simulink model "NEDC_Profiles"  (R2021b)
settings: Solver=VariableStepAuto  StartTime=0.0  StopTime=1190  RelTol=1e-3
undefined symbols (not defined in the file or in its folder): S_CYCLE, T_CYCLE, T_MAX
libraries: simulink x1
settings Model: Creator=Alireza  LastModifiedBy=Alireza

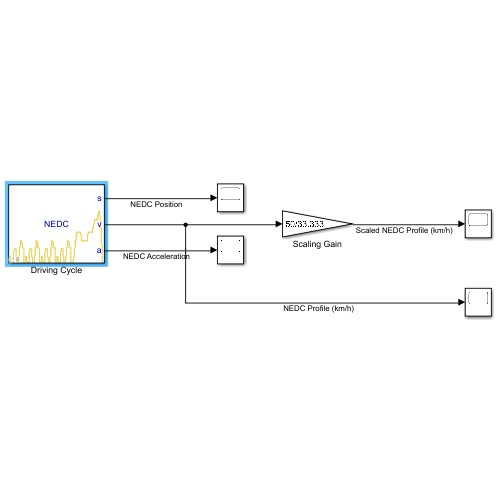
[thumbnail: Simulink's stored preview of the top-level diagram]
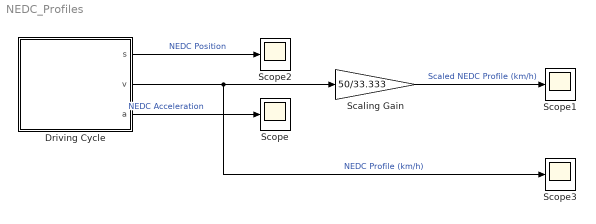
== system NEDC_Profiles ==
  Driving Cycle : Subsystem  AncestorBlock=drivingcycle_lib/Driving Cycle  mask(Driving Cycle){CycleName=NEDC, CycleRepeatsForever=off}
      mask prompts: CycleName "Cycle name:"; CycleRepeatsForever "Repeat cycle forever"
      mask help: This block produces driving cycle data, as used in many automotive applications. It outputs displacement, velocity and acceleration, all in SI units. The user can choose from a list of popular cycles.
      mask init:
      | [S_CYCLE, T_CYCLE, T_MAX, W_SCALE, Disp, Vel, Acc, t, v] = ...
      |     drivingcycleutils.maskInitFcn(CycleName, CycleRepeatsForever);
      mask Help: web(drivingcycleutils.docPath(gcb()), '-helpbrowser');
      mask TypeOptions CycleName: NEDC | ECE R15 | EUDC | ArtUrban | ArtRoad | ArtMw130 | ArtMw150 | WLTP class 3 | UDDS | FTP | HWFET
      mask Display:
      | color('yellow');
      | plot(t/max(t),3.6*v/180);
      | color('blue')
      | fprintf(CycleName);
      | port_label('output', 1, 's');
      | port_label('output', 2, 'v');
      | port_label('output', 3, 'a');
  Scaling Gain : Gain  Gain=50/33.333
  Scope{,1..3} (4 alike) : Scope
  wires:
  Driving Cycle/2(v) -> Scope3/1, Scaling Gain/1  "NEDC Profile (km/h)"
  Driving Cycle/3(a) -> Scope/1  "NEDC Acceleration"
  Scaling Gain/1 -> Scope1/1  "Scaled NEDC Profile (km/h)"
  Driving Cycle/1(s) -> Scope2/1  "NEDC Position"

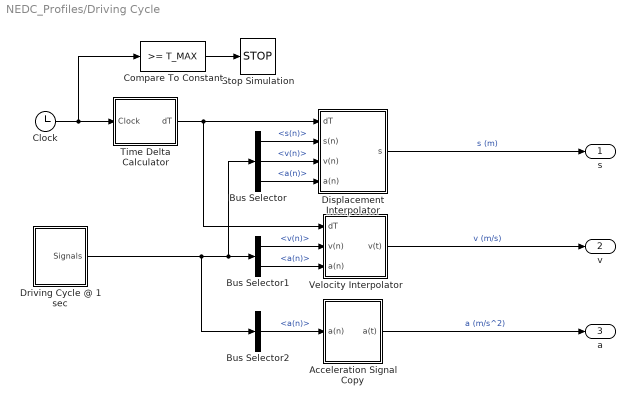
== system NEDC_Profiles/Driving Cycle ==
  Acceleration Signal Copy : Subsystem
  Bus Selector : BusSelector  OutputSignals=s(n),v(n),a(n)
  Bus Selector1 : BusSelector  OutputSignals=v(n),a(n)
  Bus Selector2 : BusSelector  OutputSignals=a(n)
  Clock : Clock
  Compare To Constant : simulink/Logic and Bit Operations/Compare To Constant  relop=>=  const=T_MAX  OutDataTypeStr=boolean
  Displacement Interpolator : Subsystem
  Driving Cycle @ 1 sec : Subsystem
  Stop Simulation : Stop
  Time Delta Calculator : Subsystem
  Velocity Interpolator : Subsystem
  s : Outport
  v : Outport  Port=2
  a : Outport  Port=3
  wires:
  Compare To Constant/1 -> Stop Simulation/1
  Time Delta Calculator/1(dT) -> Displacement Interpolator/1(dT), Velocity Interpolator/1(dT)
  Displacement Interpolator/1(s) -> s/1  "s (m)"
  Velocity Interpolator/1(v(t)) -> v/1  "v (m/s)"
  Driving Cycle @ 1 sec/1(Signals) -> Bus Selector/1, Bus Selector1/1, Bus Selector2/1
  Bus Selector/1 -> Displacement Interpolator/2(s(n))  "<s(n)>"
  Bus Selector/2 -> Displacement Interpolator/3(v(n))  "<v(n)>"
  Bus Selector/3 -> Displacement Interpolator/4(a(n))  "<a(n)>"
  Bus Selector1/1 -> Velocity Interpolator/2(v(n))  "<v(n)>"
  Bus Selector1/2 -> Velocity Interpolator/3(a(n))  "<a(n)>"
  Bus Selector2/1 -> Acceleration Signal Copy/1(a(n))  "<a(n)>"
  Acceleration Signal Copy/1(a(t)) -> a/1  "a (m/s^2)"
  Clock/1 -> Compare To Constant/1, Time Delta Calculator/1(Clock)

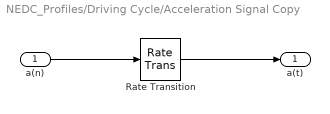
== system NEDC_Profiles/Driving Cycle/Acceleration Signal Copy ==
  a(n) : Inport
  Rate Transition : RateTransition  Integrity=off
  a(t) : Outport
  wires:
  a(n)/1 -> Rate Transition/1
  Rate Transition/1 -> a(t)/1

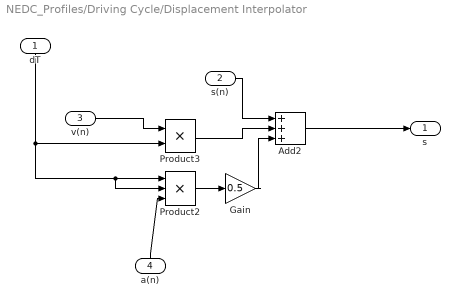
== system NEDC_Profiles/Driving Cycle/Displacement Interpolator ==
  dT : Inport
  s(n) : Inport  Port=2
  v(n) : Inport  Port=3
  a(n) : Inport  Port=4
  Add2 : Sum  Inputs=+++
  Gain : Gain  Gain=0.5
  Product2 : Product  Inputs=3  RndMeth=Zero
  Product3 : Product  RndMeth=Zero
  s : Outport
  wires:
  s(n)/1 -> Add2/1
  dT/1 -> Product3/2, Product2/2, Product2/1
  Product2/1 -> Gain/1
  Product3/1 -> Add2/2
  Add2/1 -> s/1
  Gain/1 -> Add2/3
  a(n)/1 -> Product2/3
  v(n)/1 -> Product3/1

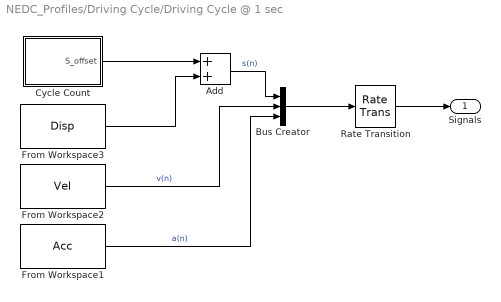
== system NEDC_Profiles/Driving Cycle/Driving Cycle @ 1 sec ==
  Add : Sum
  Bus Creator : BusCreator  Inputs=3
  Cycle Count : Subsystem
  From Workspace1 : FromWorkspace  VariableName=Acc  SampleTime=1  Interpolate=off  OutputAfterFinalValue=Cyclic repetition
  From Workspace2 : FromWorkspace  VariableName=Vel  SampleTime=1  Interpolate=off  OutputAfterFinalValue=Cyclic repetition
  From Workspace3 : FromWorkspace  VariableName=Disp  SampleTime=1  Interpolate=off  OutputAfterFinalValue=Cyclic repetition
  Rate Transition : RateTransition  Integrity=off  OutPortSampleTimeOpt=Inherit  OutPortSampleTime=SampleTime
  Signals : Outport  SampleTime=0
  wires:
  Bus Creator/1 -> Rate Transition/1
  Add/1 -> Bus Creator/1  "s(n)"
  From Workspace3/1 -> Add/2
  From Workspace2/1 -> Bus Creator/2  "v(n)"
  From Workspace1/1 -> Bus Creator/3  "a(n)"
  Cycle Count/1(S_offset) -> Add/1
  Rate Transition/1 -> Signals/1

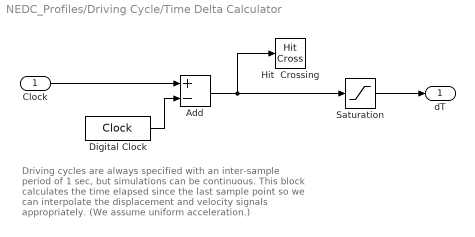
== system NEDC_Profiles/Driving Cycle/Time Delta Calculator ==
  note: Driving cycles are always specified with an inter-sample
      | period of 1 sec, but simulations can be continuous.  This
      | block calculates the time elapsed since the last sample
      | point so we can interpolate the displacement and velocity
      | signals appropriately.  (We assume uniform acceleration.)
  Clock : Inport
  Add : Sum  Inputs=+-
  Digital Clock : DigitalClock
  Hit  Crossing : HitCross  HitCrossingOffset=0.5  HitCrossingDirection=falling  ShowOutputPort=off
  Saturation : Saturate  UpperLimit=1  LowerLimit=0  ZeroCross=off
  dT : Outport
  wires:
  Digital Clock/1 -> Add/2
  Clock/1 -> Add/1
  Add/1 -> Saturation/1, Hit  Crossing/1
  Saturation/1 -> dT/1

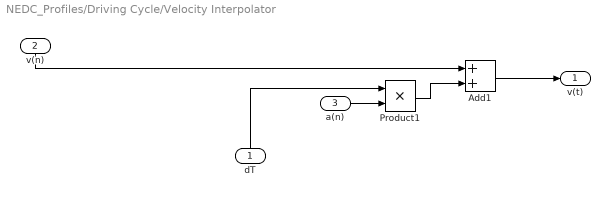
== system NEDC_Profiles/Driving Cycle/Velocity Interpolator ==
  dT : Inport
  v(n) : Inport  Port=2
  a(n) : Inport  Port=3
  Add1 : Sum
  Product1 : Product  RndMeth=Zero
  v(t) : Outport
  wires:
  Add1/1 -> v(t)/1
  a(n)/1 -> Product1/2
  v(n)/1 -> Add1/1
  dT/1 -> Product1/1
  Product1/1 -> Add1/2

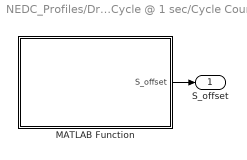
== system NEDC_Profiles/Driving Cycle/Driving Cycle @ 1 sec/Cycle Count ==
  MATLAB Function : MATLAB Function  TreatAsAtomicUnit=on
  S_offset : Outport
  wires:
  MATLAB Function/1(S_offset) -> S_offset/1

== matlab function NEDC_Profiles/Driving Cycle/Driving Cycle @ 1 sec/Cycle Count/MATLAB Function ==
  settings: updateMethod=DISCRETE  sampleTime=1
  data: S_offset output; T_CYCLE parameter; S_CYCLE parameter
function S_offset = calcDispOffset(T_CYCLE, S_CYCLE)
%#codegen

persistent sampleCount cycleCount T_CYCLE_uint32;
if isempty(cycleCount)    
    sampleCount = uint32(0);
    cycleCount  = uint32(0);
    T_CYCLE_uint32 = uint32(T_CYCLE);
end

while sampleCount >= T_CYCLE_uint32;
    cycleCount = cycleCount + uint32(1);
    sampleCount = sampleCount - T_CYCLE_uint32;
end

S_offset = S_CYCLE * double(cycleCount);

sampleCount = sampleCount + uint32(1);
end
